simulink model "VV_drive"  (R2018b)
settings: Solver=VariableStepAuto  StartTime=0.0  StopTime=10.0  RelTol=1e-3
settings Model: Creator=kekos  LastModifiedBy=kekos

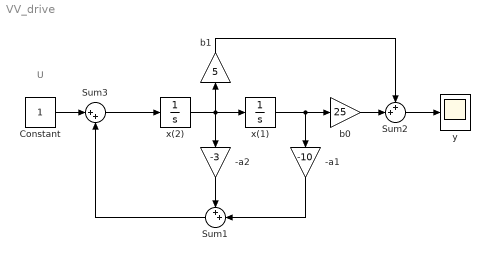
== system VV_drive ==
  note: U
  -a1 : Gain  Gain=-10
  -a2 : Gain  Gain=-3
  Constant : Constant
  Sum1 : Sum  Inputs=++|
  Sum2 : Sum  Inputs=++|
  Sum3 : Sum  Inputs=|++
  b0 : Gain  Gain=25
  b1 : Gain  Gain=5
  x(1) : Integrator  InitialCondition=3.4
  x(2) : Integrator  InitialCondition=3.4
  y : Scope
  wires:
  -a1/1 -> Sum1/2
  b1/1 -> Sum2/1
  b0/1 -> Sum2/2
  Sum2/1 -> y/1
  Sum1/1 -> Sum3/2
  -a2/1 -> Sum1/1
  x(2)/1 -> -a2/1, x(1)/1, b1/1
  x(1)/1 -> b0/1, -a1/1
  Constant/1 -> Sum3/1
  Sum3/1 -> x(2)/1
